simulink model "PMSMqidong_succeed"  (R2020b)
settings: Solver=ode15s  StartTime=0.0  StopTime=5  MaxStep=1e-5  RelTol=1e-3  EnableMultiTasking=on
libraries: powerlib x6
settings Model: Creator=84360  LastModifiedBy=ysDeng
settings DataIOCC: ReturnWorkspaceOutputs=off
settings OptimizationCC: LifeSpan=inf
settings DebuggingCC: SFUnexpectedBacktrackingDiag=warning  SFNoUnconditionalDefaultTransitionDiag=warning  ArithmeticOperatorsInVariantConditions=warning
settings SFSimCC: SimUseLocalCustomCode=off  CustomCodeUndefinedFunction=UseInterfaceOnly
settings RTWCC: RTWUseLocalCustomCode=off
settings CodeAppCC: StateflowObjectComments=on
settings GRTTargetCC: TargetLangStandard=C89/C90 (ANSI)
settings ConfigComp: CovMetricSettings=dw  CovSaveCumulativeToWorkspaceVar=on  CovSaveSingleToWorkspaceVar=on  CovExternalEMLEnable=off
settings SimscapeCC: SimscapeNormalizeSystem=off

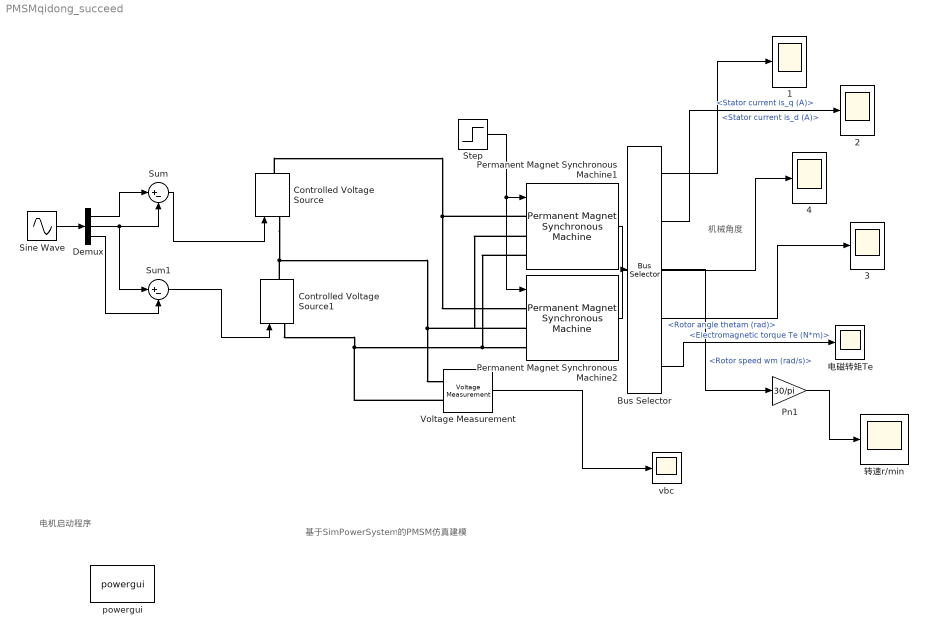
== system PMSMqidong_succeed ==
  note: 机械角度
  note: 基于SimPowerSystem的PMSM仿真建模
  note: 电机启动程序
  {1..4} (4 alike) : Scope
  Bus Selector : BusSelector  OutputSignals=Stator current is_d (A),Stator current is_q (A),Rotor speed wm (rad/s),Rotor angle thetam (rad),Electromagnetic torque Te (N*m)
  Controlled Voltage Source : powerlib/Electrical Sources/Controlled Voltage Source  Initialize=on  Source_Type=AC  Amplitude=0  Phase=0  Frequency=0  Measurements=None
  Controlled Voltage Source1 : powerlib/Electrical Sources/Controlled Voltage Source  Initialize=on  Source_Type=AC  Amplitude=0  Phase=0  Frequency=0  Measurements=None
  Demux : Demux  Outputs=3
  Permanent Magnet Synchronous Machine1 : powerlib/Machines/Permanent Magnet Synchronous Machine  NbPhases=3  FluxDistribution=Sinusoidal  RotorType=Salient-pole  MechanicalLoad=Torque Tm  PresetModel=No  ShowDetailedParameters=on  MeasurementBus=off  Resistance=11.75  Inductance=8.5e-3  dqInductances=[0.18448 0.1751]  La=0.000835  MachineConstant=Flux linkage established by magnets (V.s)  Flux=0.0372955  VoltageCst=20.294  TorqueCst=0.16783  Flat=120  Mechanical=[0.0000001 0.000303448 3]  PolePairs=4  InitialConditions=[0,0, 0,0]  InitialConditions5ph=[0 0 0 0 0 0]  RefAngle=Aligned with phase A axis (original Park)  IterativeDiscreteModel=Trapezoidal non iterative  TsBlock=-1  TsPowergui=0
  Permanent Magnet Synchronous Machine2 : powerlib/Machines/Permanent Magnet Synchronous Machine  NbPhases=3  FluxDistribution=Sinusoidal  RotorType=Salient-pole  MechanicalLoad=Torque Tm  PresetModel=No  ShowDetailedParameters=on  MeasurementBus=off  Resistance=11.75  Inductance=8.5e-3  dqInductances=[0.18448 0.1751]  La=0.000835  MachineConstant=Flux linkage established by magnets (V.s)  Flux=0.0372955  VoltageCst=20.294  TorqueCst=0.16783  Flat=120  Mechanical=[0.0000001 0.000303448 3]  PolePairs=4  InitialConditions=[0,0, 0,0]  InitialConditions5ph=[0 0 0 0 0 0]  RefAngle=Aligned with phase A axis (original Park)  IterativeDiscreteModel=Trapezoidal non iterative  TsBlock=-1  TsPowergui=0
  Pn1 : Gain  Gain=30/pi
  Sine Wave : Sin  Amplitude=200*sqrt(2)  Frequency=100*pi  Phase=[0 -2*pi/3 2*pi/3]-[-pi/2 -pi/2 -pi/2]  SampleTime=0
  Step : Step  Time=0.3  After=0  SampleTime=0
  Sum : Sum  Inputs=|+-
  Sum1 : Sum  Inputs=|+-
  Voltage Measurement : powerlib/Measurements/Voltage Measurement  PhasorSimulation=off  OutputType=Complex  PSBequivalent=0
  powergui : powerlib/powergui  Priority=1  SimulationMode=Continuous  SampleTime=50e-6  frequency=60  Iterations=50  frequencyindice=0  Pbase=100e6  ErrMax=1e-4  UnitsV=kV  UnitsW=MW  buscounter=0  FunctionMessages=off  echomessages=off  EnableUseOfTLC=off  CurrentSourceSwitches=off  DisableSnubberDevices=off  DisableRonSwitches=off  DisableVfSwitches=off  DisplayEquations=off  AutomaticDiscreteSolvers=off  SolverType=Tustin/Backward Euler (TBE)  Interpol=off  ExternalGateDelay=off  methode=off  Ts=10  x0status=blocks  SPID=off  SwTol=0  HookPort=off  NonlinearTolerance=1e-4  nMaxIteration=100  ContinueOnMaxIteration=off  RestoreLinks=warning  ResistiveCurrentMeasurement=off  Frange=[0:2:500]  Ylog=off  Xlog=on  ShowGrid=off  save=off  variable=ZData  structure=0  ZoomFFT=off  StartTime=0.0  cycles=1  DisplayStyle=1  fundamental=60  FreqAxis=off  MaxFrequency=1000  frequencyindicesteady=1  RmsSteady=1  display=off
  vbc : Scope
  电磁转矩Te : Scope
  转速r/min : Scope
  wires:
  Permanent Magnet Synchronous Machine2/1 -> Bus Selector/1
  Sum/1 -> Controlled Voltage Source/1
  Sum1/1 -> Controlled Voltage Source1/1
  Voltage Measurement/1 -> vbc/1
  Bus Selector/2 -> 2/1  "<Stator current is_q (A)>"
  Bus Selector/4 -> 3/1  "<Rotor angle thetam (rad)>"
  Bus Selector/5 -> 电磁转矩Te/1  "<Electromagnetic torque Te (N*m)>"
  Bus Selector/3 -> Pn1/1  "<Rotor speed wm (rad/s)>"
  Sine Wave/1 -> Demux/1
  Demux/1 -> Sum/1
  Demux/2 -> Sum/2, Sum1/1
  Demux/3 -> Sum1/2
  Pn1/1 -> 转速r/min/1
  Step/1 -> Permanent Magnet Synchronous Machine2/1, Permanent Magnet Synchronous Machine1/1
  Bus Selector/1 -> 1/1  "<Stator current is_d (A)>"
  Permanent Magnet Synchronous Machine1/1 -> 4/1
  connections:
  Controlled Voltage Source1/RConn1 -- Controlled Voltage Source/LConn1 -- Permanent Magnet Synchronous Machine1/LConn2 -- Permanent Magnet Synchronous Machine2/LConn2 -- Voltage Measurement/LConn1
  Controlled Voltage Source/RConn1 -- Permanent Magnet Synchronous Machine1/LConn1 -- Permanent Magnet Synchronous Machine2/LConn1
  Controlled Voltage Source1/LConn1 -- Voltage Measurement/LConn2 -- Permanent Magnet Synchronous Machine1/LConn3 -- Permanent Magnet Synchronous Machine2/LConn3
